simulink model "sunset_pv"  (R2023b)
settings: Solver=VariableStepAuto  StartTime=0.0  StopTime=10.0  RelTol=1e-3
undefined symbols (not defined in the file): Eg0, Isc, K, ki, n, Ns, q, Rs, Rsh, Tn, Voc
settings Model: Creator=camposjulca  LastModifiedBy=camposjulca

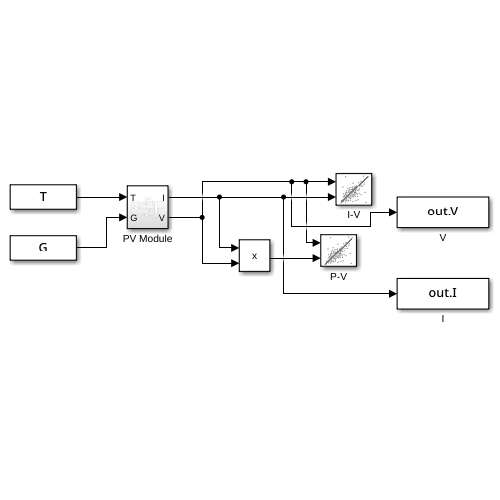
[thumbnail: Simulink's stored preview of the top-level diagram]
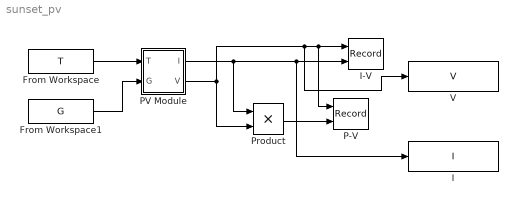
== system sunset_pv ==
  From Workspace : FromWorkspace  VariableName=T
  From Workspace1 : FromWorkspace  VariableName=G
  I : ToWorkspace  VariableName=I  SampleTime=-1
  I-V : Record  FileSettingsInternal="{\"entries\":[{\"content\":{\"excelSettings\":{\"content\":{},\"type\":\"Streamout.ExcelSettings\"}},\"type\":\"Streamout.FileSettingStorage\",\"uuid\":\"\"}],\"packageUris\":[\"http:\\/\\/schema.mathworks.com\\/mf0\\/streamout_blocks\\/R2020a\"],\"version\":\"1.0\"}"  Layout=[1 1]  SignalsInternal="{\"entries\":[{\"content\":{\"signals\":[{\"content\":{\"blockPath\":[],\"dimensions\":[1],\"domain\":\"\",\"lineColor\":\"#edb120\",\"port\":1,\"signalID\":7169,\"signalName\":\"PV Module:2\"},\"type\":\"RecordBlkView.Signal\",\"uuid\":\"\"},{\"content\":{\"blockPath\":[],\"dimensions\":[1],\"domain\":\"\",\"lineColor\":\"#7e2f8e\",\"port\":2,\"signalID\":7172,\"signalName\":\"PV Module:1\"},\"type\":\"RecordBlkView.Signal\",\"uuid\":\"\"}]},\"type\":\"RecordBlkView.InputSignals\",\"uuid\":\"\"}],\"packageUris\":[\"http:\\/\\/schema.mathworks.com\\/mf0\\/streamout_blocks\\/R2020a\"],\"version\":\"1.0\"}"  VisualizationBindings="{\"xyplotplugin\":{\"info\":[{\"series\":[],\"subplotID\":1}]}}"  CompatibilityTag=XY
  P-V : Record  FileSettingsInternal="{\"entries\":[{\"content\":{\"excelSettings\":{\"content\":{},\"type\":\"Streamout.ExcelSettings\"}},\"type\":\"Streamout.FileSettingStorage\",\"uuid\":\"\"}],\"packageUris\":[\"http:\\/\\/schema.mathworks.com\\/mf0\\/streamout_blocks\\/R2020a\"],\"version\":\"1.0\"}"  Layout=[2 1]  SignalsInternal="{\"entries\":[{\"content\":{\"signals\":[{\"content\":{\"blockPath\":[],\"dimensions\":[1],\"domain\":\"\",\"lineColor\":\"#77ac30\",\"port\":1,\"signalID\":7161,\"signalName\":\"PV Module:2\"},\"type\":\"RecordBlkView.Signal\",\"uuid\":\"\"},{\"content\":{\"blockPath\":[],\"dimensions\":[1],\"domain\":\"\",\"lineColor\":\"#4dbeee\",\"port\":2,\"signalID\":7164,\"signalName\":\"Product\"},\"type\":\"RecordBlkView.Signal\",\"uuid\":\"\"}]},\"type\":\"RecordBlkView.InputSignals\",\"uuid\":\"\"}],\"packageUris\":[\"http:\\/\\/schema.mathworks.com\\/mf0\\/streamout_blocks\\/R2020a\"],\"version\":\"1.0\"}"  VisualizationBindings="{\"xyplotplugin\":{\"info\":[{\"series\":[],\"subplotID\":1}]}}"  CompatibilityTag=XY
  PV Module : Subsystem  InitFcn=|
      | ki=0.037,
      | q=1.60217646e-19,
      | K=1.3806503e-23,
      | n=1.0,
      | Eg0=1.1,
      | Rs=0.39,
      | Rsh=545.82,
      | Tn=298,
      | Voc=47.4,
      | Isc=9.35,
      | Ns=72,
  Product : Product
  V : ToWorkspace  VariableName=V  SampleTime=-1
  wires:
  PV Module/1(I) -> Product/1, I/1, I-V/2
  PV Module/2(V) -> Product/2, V/1, P-V/1, I-V/1
  Product/1 -> P-V/2
  From Workspace/1 -> PV Module/1(T)
  From Workspace1/1 -> PV Module/2(G)

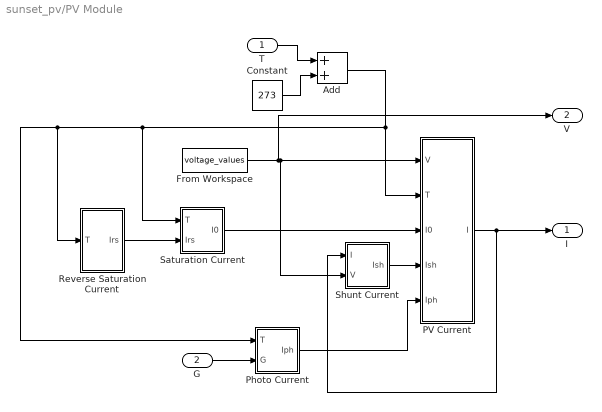
== system sunset_pv/PV Module ==
  T : Inport
  G : Inport  Port=2
  Add : Sum
  Constant : Constant  Value=273
  From Workspace : FromWorkspace  VariableName=voltage_values  OutDataTypeStr=double  SampleTime=0.1
  PV Current : Subsystem
  Photo Current : Subsystem
  Reverse Saturation Current : Subsystem
  Saturation Current : Subsystem
  Shunt Current : Subsystem
  I : Outport
  V : Outport  Port=2
  wires:
  T/1 -> Add/1
  G/1 -> Photo Current/2(G)
  Reverse Saturation Current/1(Irs) -> Saturation Current/2(Irs)
  Photo Current/1(Iph) -> PV Current/5(Iph)
  PV Current/1(I) -> I/1, Shunt Current/1(I)
  Shunt Current/1(Ish) -> PV Current/4(Ish)
  From Workspace/1 -> V/1, PV Current/1(V), Shunt Current/2(V)
  Constant/1 -> Add/2
  Saturation Current/1(I0) -> PV Current/3(I0)
  Add/1 -> Saturation Current/1(T), Reverse Saturation Current/1(T), Photo Current/1(T), PV Current/2(T)

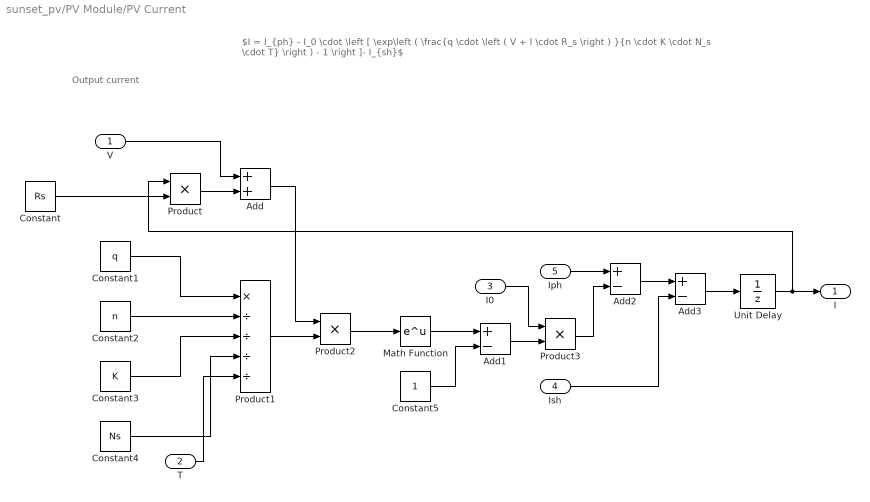
== system sunset_pv/PV Module/PV Current ==
  note: $I = I_{ph} - I_0 \cdot \left [ \exp\left ( \frac{q \cdot \left ( V + I \cdot R_s \right ) }{n \cdot K \cdot N_s \cdot T} \right ) - 1 \right ]- I_{sh}$
  note: Output current
  V : Inport
  T : Inport  Port=2
  I0 : Inport  Port=3
  Ish : Inport  Port=4
  Iph : Inport  Port=5
  Add : Sum
  Add1 : Sum  Inputs=+-
  Add2 : Sum  Inputs=+-
  Add3 : Sum  Inputs=+-
  Constant : Constant  Value=Rs
  Constant1 : Constant  Value=q
  Constant2 : Constant  Value=n
  Constant3 : Constant  Value=K
  Constant4 : Constant  Value=Ns
  Constant5 : Constant
  Math Function : Math
  Product : Product
  Product1 : Product  Inputs=*////
  Product2 : Product
  Product3 : Product
  Unit Delay : UnitDelay  SampleTime=-1  HasFrameUpgradeWarning=on
  I : Outport
  wires:
  Constant5/1 -> Add1/2
  Product2/1 -> Math Function/1
  Product1/1 -> Product2/2
  Product3/1 -> Add2/2
  Product/1 -> Add/2
  V/1 -> Add/1
  Constant4/1 -> Product1/4
  Constant/1 -> Product/2
  Math Function/1 -> Add1/1
  Constant1/1 -> Product1/1
  Constant3/1 -> Product1/3
  Add2/1 -> Add3/1
  I0/1 -> Product3/1
  T/1 -> Product1/5
  Add1/1 -> Product3/2
  Constant2/1 -> Product1/2
  Add/1 -> Product2/1
  Iph/1 -> Add2/1
  Add3/1 -> Unit Delay/1
  Ish/1 -> Add3/2
  Unit Delay/1 -> Product/1, I/1

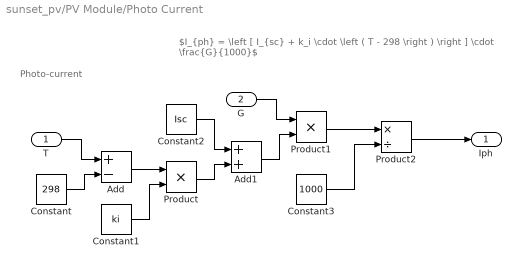
== system sunset_pv/PV Module/Photo Current ==
  note: Photo-current
  note: $I_{ph} = \left [ I_{sc} + k_i \cdot \left ( T - 298 \right ) \right ] \cdot \frac{G}{1000}$
  T : Inport
  G : Inport  Port=2
  Add : Sum  Inputs=+-
  Add1 : Sum
  Constant : Constant  Value=298
  Constant1 : Constant  Value=ki
  Constant2 : Constant  Value=Isc
  Constant3 : Constant  Value=1000
  Product : Product
  Product1 : Product
  Product2 : Product  Inputs=*/
  Iph : Outport
  wires:
  Add/1 -> Product/1
  Product/1 -> Add1/2
  T/1 -> Add/1
  Add1/1 -> Product1/2
  Constant3/1 -> Product2/2
  Product2/1 -> Iph/1
  Constant1/1 -> Product/2
  Product1/1 -> Product2/1
  Constant/1 -> Add/2
  Constant2/1 -> Add1/1
  G/1 -> Product1/1

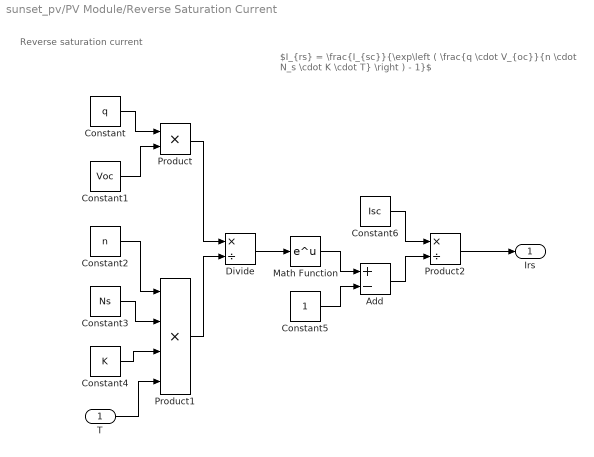
== system sunset_pv/PV Module/Reverse Saturation Current ==
  note: Reverse saturation current
  note: $I_{rs} = \frac{I_{sc}}{\exp\left ( \frac{q \cdot V_{oc}}{n \cdot N_s \cdot K \cdot T} \right ) - 1}$
  T : Inport
  Add : Sum  Inputs=+-
  Constant : Constant  Value=q
  Constant1 : Constant  Value=Voc
  Constant2 : Constant  Value=n
  Constant3 : Constant  Value=Ns
  Constant4 : Constant  Value=K
  Constant5 : Constant
  Constant6 : Constant  Value=Isc
  Divide : Product  Inputs=*/
  Math Function : Math
  Product : Product
  Product1 : Product  Inputs=4
  Product2 : Product  Inputs=*/
  Irs : Outport
  wires:
  Constant/1 -> Product/1
  Constant4/1 -> Product1/3
  Add/1 -> Product2/2
  T/1 -> Product1/4
  Constant6/1 -> Product2/1
  Product1/1 -> Divide/2
  Constant5/1 -> Add/2
  Constant3/1 -> Product1/2
  Product2/1 -> Irs/1
  Math Function/1 -> Add/1
  Constant2/1 -> Product1/1
  Constant1/1 -> Product/2
  Divide/1 -> Math Function/1
  Product/1 -> Divide/1

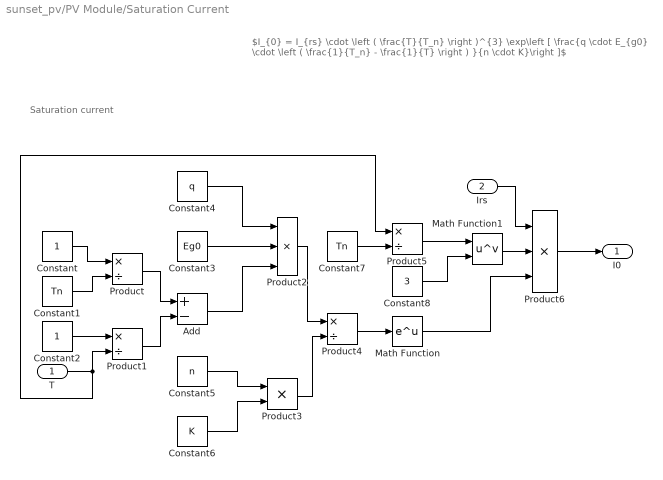
== system sunset_pv/PV Module/Saturation Current ==
  note: Saturation current
  note: $I_{0} = I_{rs} \cdot \left ( \frac{T}{T_n} \right )^{3} \exp\left [ \frac{q \cdot E_{g0} \cdot \left ( \frac{1}{T_n} - \frac{1}{T} \right ) }{n \cdot K}\right ]$
  T : Inport
  Irs : Inport  Port=2
  Add : Sum  Inputs=+-
  Constant : Constant
  Constant1 : Constant  Value=Tn
  Constant2 : Constant
  Constant3 : Constant  Value=Eg0
  Constant4 : Constant  Value=q
  Constant5 : Constant  Value=n
  Constant6 : Constant  Value=K
  Constant7 : Constant  Value=Tn
  Constant8 : Constant  Value=3
  Math Function : Math
  Math Function1 : Math  Operator=pow
  Product{,1,4..5} (4 alike) : Product  Inputs=*/
  Product2 : Product  Inputs=***
  Product3 : Product
  Product6 : Product  Inputs=3
  I0 : Outport
  wires:
  Math Function1/1 -> Product6/2
  Constant/1 -> Product/1
  Constant3/1 -> Product2/2
  Constant7/1 -> Product5/2
  Product3/1 -> Product4/2
  Constant8/1 -> Math Function1/2
  Product6/1 -> I0/1
  T/1 -> Product1/2, Product5/1
  Constant2/1 -> Product1/1
  Add/1 -> Product2/3
  Product2/1 -> Product4/1
  Product1/1 -> Add/2
  Constant4/1 -> Product2/1
  Product/1 -> Add/1
  Math Function/1 -> Product6/3
  Product5/1 -> Math Function1/1
  Irs/1 -> Product6/1
  Constant1/1 -> Product/2
  Product4/1 -> Math Function/1
  Constant6/1 -> Product3/2
  Constant5/1 -> Product3/1

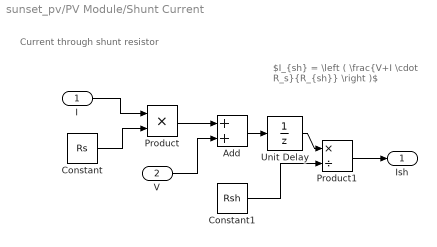
== system sunset_pv/PV Module/Shunt Current ==
  note: Current through shunt resistor
  note: $I_{sh} = \left ( \frac{V+I \cdot R_s}{R_{sh}} \right )$
  I : Inport
  V : Inport  Port=2
  Add : Sum
  Constant : Constant  Value=Rs
  Constant1 : Constant  Value=Rsh
  Product : Product
  Product1 : Product  Inputs=*/
  Unit Delay : UnitDelay  SampleTime=-1  HasFrameUpgradeWarning=on
  Ish : Outport
  wires:
  Constant/1 -> Product/2
  Constant1/1 -> Product1/2
  Product/1 -> Add/1
  V/1 -> Add/2
  I/1 -> Product/1
  Product1/1 -> Ish/1
  Add/1 -> Unit Delay/1
  Unit Delay/1 -> Product1/1
